simulink library "MPSV"  (R2025b)
settings: Solver=VariableStepAuto  StartTime=0.0  StopTime=10.0  RelTol=1e-3
undefined symbols (not defined in the file or in its folder): cost, errorCode, goalReached, isFeasible, numberOfPerformedIterations, numPoses, outOfNodes, path, timestampOfComputationUTC
libraries: simulink x31, $bdroot x11, etargetslib x5
(part 1 of 3)
settings Model: Creator=damerius  LastModifiedBy=damerius
settings SolverCC: AlgebraicLoopSolver=TrustRegion
settings OptimizationCC: ReuseModelBlockBuffer=off
settings DebuggingCC: UnconnectedInputMsg=warning  UnconnectedOutputMsg=warning  UnconnectedLineMsg=warning
settings ModelReferenceCC: EnableRefExpFcnMdlSchedulingChecks=on
settings RTWCC: GPUComputeCapability=3.5  DLArmComputeVersion=19.05

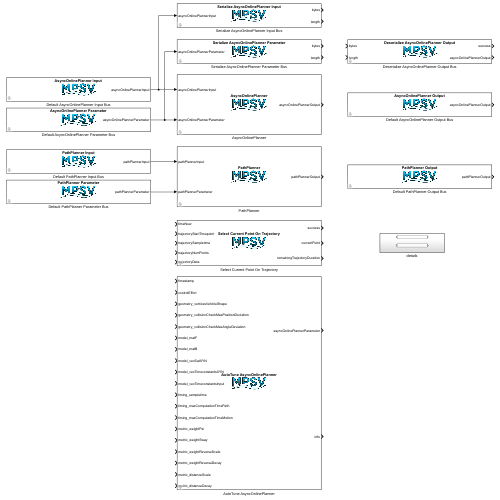
[thumbnail: Simulink's stored preview of the top-level diagram]
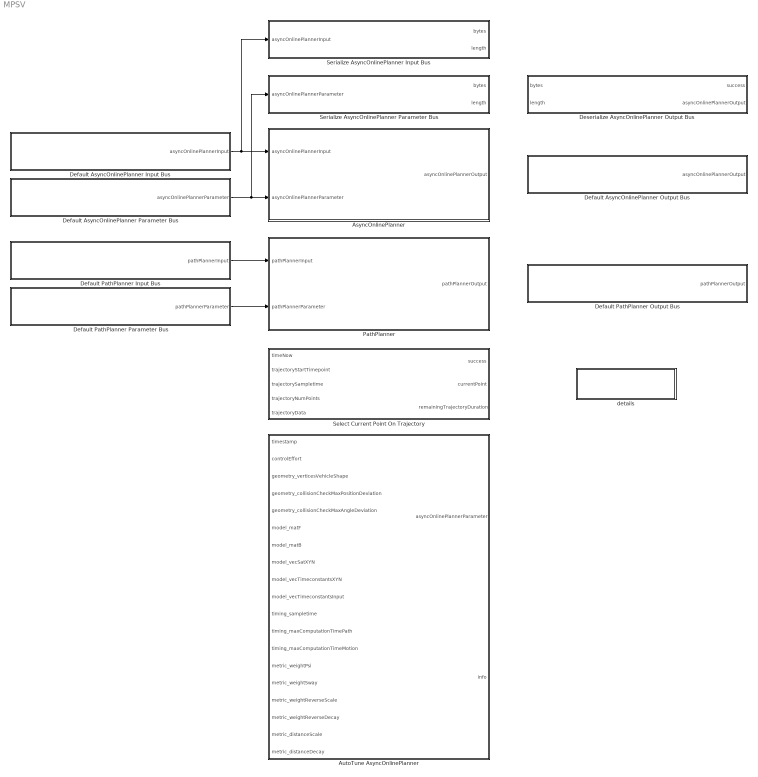
== system MPSV ==
  AsyncOnlinePlanner : Subsystem  mask{pathMaxNumNodes=200, pathMaxNumSamples=1000000, motionMaxNumNodes=200, motionMaxNumSamples=1000000, threadPriority=20, cpuCoreIDs=[], ompNumThreads=-1, ompDynamic=-1}
      mask prompts: pathMaxNumNodes "Maximum number of nodes for path planning (at least 2):"; pathMaxNumSamples "Maximum number of samples for path planning (at least 1):"; motionMaxNumNodes "Maximum number of nodes for motion planning (at least 2):"; motionMaxNumSamples "Maximum number of samples for path planning (at least 1):"; threadPriority "Thread priority (1: low, 99: high):"; cpuCoreIDs "CPU cores on which the thread is eligible to run, e.g. [0,1,2,3] ([] to ignore):"; ompNumThreads "OMP_NUM_THREADS (less than 1 to ignore):"; ompDynamic "OMP_DYNAMIC (-1 to ignore):"
      mask help:
      | Solve the online sequential motion planning problem in an asynchronous running parallel thread. For all kinds of timestamps, an arbitrary time source can be selected by the user. However, all times must be given in seconds and must be monotonically increasing.<br><br>
      |
      | <b>threadState</b><br>
      | The execution state of the asynchronous thread has the following enumeration:<br>
      | <table border="1" cellpadding="4" cellspacing="2">
      | <tr><th align="left">Value</th><th align="left">Name</th><th align="left">Description</th></tr>
      | <tr><td>0</td><td>offline</td><td>Thread has not been started.</td></tr>
      | <tr><td>1</td><td>standby</td><td>Thread is suspended and waits forever.</td></tr>
      | <tr><td>2</td><td>running</td><td>Thread solves motion planning problem.</td></tr>
      | </table>
      mask Help: eval('mpsv.OpenDocumentation(''library_asynconlineplanner.html'');');
      mask DialogControl DescGroupVar Prompt: MPSV - AsyncOnlinePlanner
      mask DialogControl Container4 Prompt: Memory Settings
      mask DialogControl Container2 Prompt: Path Planner
      mask DialogControl Container5 Prompt: Motion Planner
      mask DialogControl Container6 Prompt: Thread Settings
      mask DialogControl Container7 Prompt: Parallel Computing
      mask Display:
      | % Get dimension of block
      | pos = get_param(gcb, 'Position');
      | width = pos(3) - pos(1);
      | height = pos(4) - pos(2);
      | 
      | % Set image to center of block
      | imgWidth = 93;
      | imgHeight = 32;
      | image('MPSV_Icon.svg', [0.5*(width-imgWidth),0.5*(height-imgHeight),imgWidth,imgHeight]);
      | 
      | % Block title
      | text(0.5*width,0.5*(height+imgHeight)+2, '{\bfAsyncOnlinePlanner}','horizontalAlignment','center','verticalAlignment','bottom','texmode','on');
  AutoTune AsyncOnlinePlanner : Subsystem  mask{timeoutInput=1, periodGoalSampling=30}
      mask prompts: timeoutInput "Timeout for input data to the solver (default is 1):"; periodGoalSampling "Goal sampling period (default is 30):"
      mask help:
      | Calculate all tuning parameters for the MPSV AsyncOnlinePlanner based on given vehicle parameters and one intuitive tuning parameter. For more information take a look to the help page of mpsv.designer.AutoTune.<br><br>
      | <b>timestamp</b><br>
      | The timestamp to be set for the parameter data whenever at least one parameter changes.<br><br>
      | <b>controlEffort</b><br>
      | The amount of control effort in range (0,1] used to drive the vehicle in a steady-state in longitudinal direction.<br>
      mask DialogControl DescGroupVar Prompt: MPSV - AutoTune AsyncOnlinePlanner
      mask Display:
      | % Get dimension of block
      | pos = get_param(gcb, 'Position');
      | width = pos(3) - pos(1);
      | height = pos(4) - pos(2);
      | 
      | % Set image to center of block
      | imgWidth = 93;
      | imgHeight = 32;
      | image('MPSV_Icon.svg', [0.5*(width-imgWidth),0.5*(height-imgHeight),imgWidth,imgHeight]);
      | 
      | % Block title
      | text(0.5*width,0.5*(height+imgHeight)+2, '{\bfAutoTune AsyncOnlinePlanner}','horizontalAlignment','center','verticalAlignment','bottom','texmode','on');
  Default AsyncOnlinePlanner Input Bus : Subsystem
      mask help: Construct a default input bus for the AsyncOnlinePlanner. All values are set to zero.
      mask Help: eval('mpsv.OpenDocumentation(''library_asynconlineplannerinput.html'');');
      mask DialogControl DescGroupVar Prompt: MPSV - Default AsyncOnlinePlanner Input Bus
      mask Display:
      | % Get dimension of block
      | pos = get_param(gcb, 'Position');
      | width = pos(3) - pos(1);
      | height = pos(4) - pos(2);
      | 
      | % Set image to center of block
      | imgWidth = 93;
      | imgHeight = 32;
      | image('MPSV_Icon.svg', [0.5*(width-imgWidth),0.5*(height-imgHeight),imgWidth,imgHeight]);
      | 
      | % Block title
      | text(0.5*width,0.5*(height+imgHeight)+2, '{\bfAsyncOnlinePlanner Input}','horizontalAlignment','center','verticalAlignment','bottom','texmode','on');
  Default AsyncOnlinePlanner Output Bus : Subsystem
      mask help: Construct a default output bus for the AsyncOnlinePlanner. All values are set to zero.
      mask Help: eval('mpsv.OpenDocumentation(''library_asynconlineplanneroutput.html'');');
      mask DialogControl DescGroupVar Prompt: MPSV - Default AsyncOnlinePlanner Output Bus
      mask Display:
      | % Get dimension of block
      | pos = get_param(gcb, 'Position');
      | width = pos(3) - pos(1);
      | height = pos(4) - pos(2);
      | 
      | % Set image to center of block
      | imgWidth = 93;
      | imgHeight = 32;
      | image('MPSV_Icon.svg', [0.5*(width-imgWidth),0.5*(height-imgHeight),imgWidth,imgHeight]);
      | 
      | % Block title
      | text(0.5*width,0.5*(height+imgHeight)+2, '{\bfAsyncOnlinePlanner Output}','horizontalAlignment','center','verticalAlignment','bottom','texmode','on');
  Default AsyncOnlinePlanner Parameter Bus : Subsystem
      mask help: Construct a default parameter bus for the AsyncOnlinePlanner. All values are set to valid default values.
      mask Help: eval('mpsv.OpenDocumentation(''library_asynconlineplannerparameter.html'');');
      mask DialogControl DescGroupVar Prompt: MPSV - Default AsyncOnlinePlanner Parameter Bus
      mask Display:
      | % Get dimension of block
      | pos = get_param(gcb, 'Position');
      | width = pos(3) - pos(1);
      | height = pos(4) - pos(2);
      | 
      | % Set image to center of block
      | imgWidth = 93;
      | imgHeight = 32;
      | image('MPSV_Icon.svg', [0.5*(width-imgWidth),0.5*(height-imgHeight),imgWidth,imgHeight]);
      | 
      | % Block title
      | text(0.5*width,0.5*(height+imgHeight)+2, '{\bfAsyncOnlinePlanner Parameter}','horizontalAlignment','center','verticalAlignment','bottom','texmode','on');
  Default PathPlanner Input Bus : Subsystem
      mask help: Construct a default input bus for the PathPlanner. All values are set to zero.
      mask Help: eval('mpsv.OpenDocumentation(''library_pathplannerinput.html'');');
      mask DialogControl DescGroupVar Prompt: MPSV - Default PathPlanner Input Bus
      mask Display:
      | % Get dimension of block
      | pos = get_param(gcb, 'Position');
      | width = pos(3) - pos(1);
      | height = pos(4) - pos(2);
      | 
      | % Set image to center of block
      | imgWidth = 93;
      | imgHeight = 32;
      | image('MPSV_Icon.svg', [0.5*(width-imgWidth),0.5*(height-imgHeight),imgWidth,imgHeight]);
      | 
      | % Block title
      | text(0.5*width,0.5*(height+imgHeight)+2, '{\bfPathPlanner Input}','horizontalAlignment','center','verticalAlignment','bottom','texmode','on');
  Default PathPlanner Output Bus : Subsystem
      mask help: Construct a default output bus for the PathPlanner. All values are set to zero.
      mask Help: eval('mpsv.OpenDocumentation(''library_pathplanneroutput.html'');');
      mask DialogControl DescGroupVar Prompt: MPSV - Default PathPlanner Output Bus
      mask Display:
      | % Get dimension of block
      | pos = get_param(gcb, 'Position');
      | width = pos(3) - pos(1);
      | height = pos(4) - pos(2);
      | 
      | % Set image to center of block
      | imgWidth = 93;
      | imgHeight = 32;
      | image('MPSV_Icon.svg', [0.5*(width-imgWidth),0.5*(height-imgHeight),imgWidth,imgHeight]);
      | 
      | % Block title
      | text(0.5*width,0.5*(height+imgHeight)+2, '{\bfPathPlanner Output}','horizontalAlignment','center','verticalAlignment','bottom','texmode','on');
  Default PathPlanner Parameter Bus : Subsystem
      mask help: Construct a default parameter bus for the PathPlanner. All values are set to valid default values.
      mask Help: eval('mpsv.OpenDocumentation(''library_pathplannerparameter.html'');');
      mask DialogControl DescGroupVar Prompt: MPSV - Default PathPlanner Parameter Bus
      mask Display:
      | % Get dimension of block
      | pos = get_param(gcb, 'Position');
      | width = pos(3) - pos(1);
      | height = pos(4) - pos(2);
      | 
      | % Set image to center of block
      | imgWidth = 93;
      | imgHeight = 32;
      | image('MPSV_Icon.svg', [0.5*(width-imgWidth),0.5*(height-imgHeight),imgWidth,imgHeight]);
      | 
      | % Block title
      | text(0.5*width,0.5*(height+imgHeight)+2, '{\bfPathPlanner Parameter}','horizontalAlignment','center','verticalAlignment','bottom','texmode','on');
  Deserialize AsyncOnlinePlanner Output Bus : Subsystem
      mask help: Deserialize an AsyncOnlinePlanner output bus from a binary representation.
      mask Help: eval('mpsv.OpenDocumentation(''library_deserializeasynconlineplanneroutput.html'');');
      mask DialogControl DescGroupVar Prompt: MPSV - Deserialize AsyncOnlinePlanner Output Bus
      mask Display:
      | % Get dimension of block
      | pos = get_param(gcb, 'Position');
      | width = pos(3) - pos(1);
      | height = pos(4) - pos(2);
      | 
      | % Set image to center of block
      | imgWidth = 93;
      | imgHeight = 32;
      | image('MPSV_Icon.svg', [0.5*(width-imgWidth),0.5*(height-imgHeight),imgWidth,imgHeight]);
      | 
      | % Block title
      | text(0.5*width,0.5*(height+imgHeight)+2, '{\bfDeserialize AsyncOnlinePlanner Output}','horizontalAlignment','center','verticalAlignment','bottom','texmode','on');
  PathPlanner : Subsystem  mask{maxNumNodes=200, maxNumSamples=1000000}
      mask prompts: maxNumNodes "Maximum number of nodes (at least 2):"; maxNumSamples "Maximum number of samples (at least 1):"
      mask help: Solve the path planning problem. The computation time to be used by the planner is set via the parameter input. For all kinds of timestamps, an arbitrary time source can be selected by the user. However, all times must be given in seconds and must be monotonically increasing.
      mask Help: eval('mpsv.OpenDocumentation(''library_pathplanner.html'');');
      mask DialogControl DescGroupVar Prompt: Path Planner
      mask DialogControl ParameterGroupVar Prompt: Memory Settings
      mask Display:
      | % Get dimension of block
      | pos = get_param(gcb, 'Position');
      | width = pos(3) - pos(1);
      | height = pos(4) - pos(2);
      | 
      | % Set image to center of block
      | imgWidth = 93;
      | imgHeight = 32;
      | image('MPSV_Icon.svg', [0.5*(width-imgWidth),0.5*(height-imgHeight),imgWidth,imgHeight]);
      | 
      | % Block title
      | text(0.5*width,0.5*(height+imgHeight)+2, '{\bfPathPlanner}','horizontalAlignment','center','verticalAlignment','bottom','texmode','on');
  Select Current Point On Trajectory : Subsystem
      mask help:
      | Select the current point on a given trajectory for a given timepoint. An arbitrary time source can be selected by the user. However, all times must be given in seconds and must be monotonically increasing.<br><br>
      |
      | <b>timeNow</b><br>
      | The current timepoint to be used to query the point on the given trajectory.
      | <br><br>
      |
      | <b>trajectoryStartTimepoint</b><br>
      | The timepoint that indicates the first data point of the trajectory.
      | <br><br>
      |
      | <b>trajectorySampletime</b><br>
      | The temporal distance between two points of the trajectory.
      | <br><br>
      |
      | <b>trajectoryNumPoints</b><br>
      | The number of points to be considered from the trajectoryData matrix.
      | <br><br>
      |
      | <b>trajectoryData</b><br>
      | A 12-by-500 matrix containing 500 points of the trajectory, where each point represents the state-input-vector [x; y; psi; u; v; r; X; Y; N; Xc; Yc; Nc].
      | <br><br>
      |
      | <b>success</b><br>
      | True if timeNow lies within the temporal range of the trajectory and a point can be selected, false otherwise.
      | <br><br>
      |
      | <b>currentPoint</b><br>
      | A bus containing the linear interpolated state values and the zero-order hold input values.
      | <br><br>
      |
      | <b>remainingTrajectoryDuration</b><br>
      | Time from timeNow to the end of the trajectory.
      mask Help: eval('mpsv.OpenDocumentation(''library_selectcurrentpointontrajectory.html'');');
      mask DialogControl DescGroupVar Prompt: MPSV - Select Current Point On Trajectory
      mask Display:
      | % Get dimension of block
      | pos = get_param(gcb, 'Position');
      | width = pos(3) - pos(1);
      | height = pos(4) - pos(2);
      | 
      | % Set image to center of block
      | imgWidth = 93;
      | imgHeight = 32;
      | image('MPSV_Icon.svg', [0.5*(width-imgWidth),0.5*(height-imgHeight),imgWidth,imgHeight]);
      | 
      | % Block title
      | text(0.5*width,0.5*(height+imgHeight)+2, '{\bfSelect Current Point On Trajectory}','horizontalAlignment','center','verticalAlignment','bottom','texmode','on');
  Serialize AsyncOnlinePlanner Input Bus : Subsystem
      mask help: Serialize an AsyncOnlinePlanner input bus to a binary representation.
      mask Help: eval('mpsv.OpenDocumentation(''library_serializeasynconlineplannerinput.html'');');
      mask DialogControl DescGroupVar Prompt: MPSV - Serialize AsyncOnlinePlanner Input Bus
      mask Display:
      | % Get dimension of block
      | pos = get_param(gcb, 'Position');
      | width = pos(3) - pos(1);
      | height = pos(4) - pos(2);
      | 
      | % Set image to center of block
      | imgWidth = 93;
      | imgHeight = 32;
      | image('MPSV_Icon.svg', [0.5*(width-imgWidth),0.5*(height-imgHeight),imgWidth,imgHeight]);
      | 
      | % Block title
      | text(0.5*width,0.5*(height+imgHeight)+2, '{\bfSerialize AsyncOnlinePlanner Input}','horizontalAlignment','center','verticalAlignment','bottom','texmode','on');
  Serialize AsyncOnlinePlanner Parameter Bus : Subsystem
      mask help: Serialize an AsyncOnlinePlanner parameter bus to a binary representation.
      mask Help: eval('mpsv.OpenDocumentation(''library_serializeasynconlineplannerparameter.html'');');
      mask DialogControl DescGroupVar Prompt: MPSV - Serialize AsyncOnlinePlanner Parameter Bus
      mask Display:
      | % Get dimension of block
      | pos = get_param(gcb, 'Position');
      | width = pos(3) - pos(1);
      | height = pos(4) - pos(2);
      | 
      | % Set image to center of block
      | imgWidth = 93;
      | imgHeight = 32;
      | image('MPSV_Icon.svg', [0.5*(width-imgWidth),0.5*(height-imgHeight),imgWidth,imgHeight]);
      | 
      | % Block title
      | text(0.5*width,0.5*(height+imgHeight)+2, '{\bfSerialize AsyncOnlinePlanner Parameter}','horizontalAlignment','center','verticalAlignment','bottom','texmode','on');
  details : Subsystem
  wires:
  Default PathPlanner Input Bus/1(pathPlannerInput) -> PathPlanner/1(pathPlannerInput)
  Default AsyncOnlinePlanner Input Bus/1(asyncOnlinePlannerInput) -> Serialize AsyncOnlinePlanner Input Bus/1(asyncOnlinePlannerInput), AsyncOnlinePlanner/1(asyncOnlinePlannerInput)
  Default AsyncOnlinePlanner Parameter Bus/1(asyncOnlinePlannerParameter) -> Serialize AsyncOnlinePlanner Parameter Bus/1(asyncOnlinePlannerParameter), AsyncOnlinePlanner/2(asyncOnlinePlannerParameter)
  Default PathPlanner Parameter Bus/1(pathPlannerParameter) -> PathPlanner/2(pathPlannerParameter)

== system MPSV/AsyncOnlinePlanner ==
  asyncOnlinePlannerInput : Inport
  asyncOnlinePlannerParameter : Inport  Port=2
  Deserialize AsyncOnlinePlanner Output Bus : $bdroot/Deserialize AsyncOnlinePlanner Output Bus
  SFunctionMPSVAsynchronousOnlinePlanner : S-Function  FunctionName=SFunctionMPSVAsynchronousOnlinePlanner  Parameters=SParameter1, SParameter2, SParameter3, SParameter4, SParameter5, SParameter6, SParameter7, SParameter8, SParameter9  SFunctionDeploymentMode=off  EnableBusSupport=off  mask(Legacy Function){SFunctionSpec=void MPSV_AsynchronousOnlinePlannerStep(void* work1, uint8 y1[52907], uint8 u1[64193], uint8 u2[1917]), SParameter1=int16(pathMaxNumNodes), SParameter2=uint32(pathMaxNumSamples), SParameter3=int16(motionMaxNumNodes), SParameter4=uint32(motionMaxNumSamples), SParameter5=int32(threadPriority), SParameter6=int32(ompNumThreads), SParameter7=int32(ompDynamic), SParameter8=int32([reshape(cpuCoreIDs,[],1); -1]), SParameter9=uint32(numel(cpuCoreIDs)), ShowSpec=on}
      mask prompts: SParameter1 "P1:"; SParameter2 "P2:"; SParameter3 "P3:"; SParameter4 "P4:"; SParameter5 "P5:"; SParameter6 "P6:"; SParameter7 "P7:"; SParameter8 "P8:"; SParameter9 "P9:"; ShowSpec "Display function specification"
      mask help:
      | This block allows you to call the legacy functions specified by the following Legacy Code Tool definition:
      | def.SFunctionName = 'SFunctionMPSVAsynchronousOnlinePlanner';
      | def.OutputFcnSpec = 'void MPSV_AsynchronousOnlinePlannerStep(void* work1, uint8 y1[52907], uint8 u1[64193], uint8 u2[1917])';
      | def.StartFcnSpec = 'void MPSV_AsynchronousOnlinePlannerInitialize(void** work1, int16 p1, uint32 p2, int16 p3, uint32 p4, int32 p5, int32 p6, int32 p7, int32 p8[], uint32 p9)';
      | def.TerminateFcnSpec = 'void MPSV_AsynchronousOnlinePlannerTerminate(void* work1)';
      | def.HeaderFiles = {'MPSV_DriverAsynchronousOnlinePlanner.hpp'};
      | def.SourceFiles = {'MPSV_DriverAsynchronousOnlinePlanner.cpp', 'MPSV_WrapperAsynchronousOnlinePlanner.cpp'};
      | def.IncPaths = {'code'};
      | def.SrcPaths = {'code'};
      | def.Options.useTlcWithAccel = false;
      mask Help: <p>This block was generated automatically by the Legacy Code Tool. For detailed help on this tool, call<a href="matlab:legacy_code('help')"> legacy_code('help')</a>.</p>
      mask Callback ShowSpec:
      | if strcmp(get_param(gcbh, 'ShowSpec'), 'on')
      |   set_param(gcbh, 'MaskDisplay', sprintf('fprintf(''%s'');', get_param(gcbh, 'SFunctionSpec')));
      | else
      |   set_param(gcbh, 'MaskDisplay', sprintf('fprintf(''%s'');', get_param(gcbh, 'FunctionName')));
      | end
      mask Display: fprintf('void MPSV_AsynchronousOnlinePlannerStep(void* work1, uint8 y1[52907], uint8 u1[64193], uint8 u2[1917])');
  Serialize AsyncOnlinePlanner Input Bus : $bdroot/Serialize AsyncOnlinePlanner Input Bus
  Serialize AsyncOnlinePlanner Parameter Bus : $bdroot/Serialize AsyncOnlinePlanner Parameter Bus
  Terminator : Terminator
  Terminator1 : Terminator
  Terminator2 : Terminator
  Width : Width  DataType=uint32
  asyncOnlinePlannerOutput : Outport
  wires:
  asyncOnlinePlannerInput/1 -> Serialize AsyncOnlinePlanner Input Bus/1
  Deserialize AsyncOnlinePlanner Output Bus/2 -> asyncOnlinePlannerOutput/1
  asyncOnlinePlannerParameter/1 -> Serialize AsyncOnlinePlanner Parameter Bus/1
  SFunctionMPSVAsynchronousOnlinePlanner/1 -> Width/1, Deserialize AsyncOnlinePlanner Output Bus/1
  Serialize AsyncOnlinePlanner Input Bus/1 -> SFunctionMPSVAsynchronousOnlinePlanner/1
  Serialize AsyncOnlinePlanner Parameter Bus/1 -> SFunctionMPSVAsynchronousOnlinePlanner/2
  Serialize AsyncOnlinePlanner Input Bus/2 -> Terminator/1
  Serialize AsyncOnlinePlanner Parameter Bus/2 -> Terminator1/1
  Width/1 -> Deserialize AsyncOnlinePlanner Output Bus/2
  Deserialize AsyncOnlinePlanner Output Bus/1 -> Terminator2/1

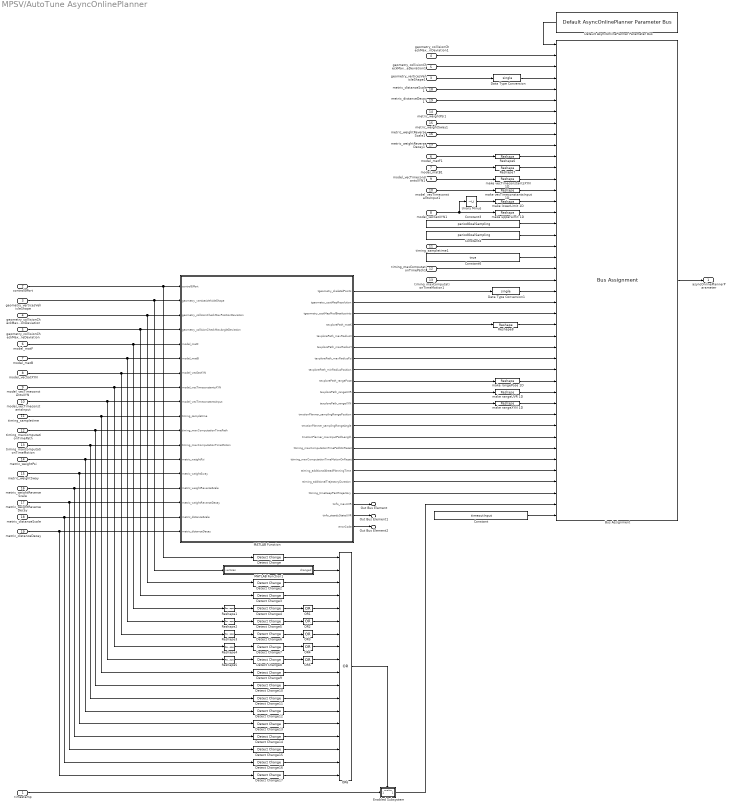
== system MPSV/AutoTune AsyncOnlinePlanner ==
  timestamp : Inport
  controlEffort : Inport  Port=2
  geometry_verticesVehicleShape : Inport  Port=3
  geometry_collisionCheckMaxPositionDeviation : Inport  Port=4
  geometry_collisionCheckMaxAngleDeviation : Inport  Port=5
  model_matF : Inport  Port=6
  model_matB : Inport  Port=7
  model_vecSatXYN : Inport  Port=8
  model_vecTimeconstantsXYN : Inport  Port=9
  model_vecTimeconstantsInput : Inport  Port=10
  timing_sampletime : Inport  Port=11
  timing_maxComputationTimePath : Inport  Port=12
  timing_maxComputationTimeMotion : Inport  Port=13
  metric_weightPsi : Inport  Port=14
  metric_weightSway : Inport  Port=15
  metric_weightReverseScale : Inport  Port=16
  metric_weightReverseDecay : Inport  Port=17
  metric_distanceScale : Inport  Port=18
  metric_distanceDecay : Inport  Port=19
  Bus Assignment : BusAssignment  AssignedSignals=sequentialPlanner.geometry.collisionCheckMaxPositionDeviation,sequentialPlanner.geometry.collisionCheckMaxAngleDeviation,sequentialPlanner.geometry.verticesVehicleShape,sequentialPlanner.costMap.distanceScale,sequentialPlanner.costMap.distanceDecay,sequentialPlanner.metric.weightPsi,sequentialPlanner.metric.weightSway,sequentialPlanner.metric.weightReverseScale,sequentialPlanner.metric.weightReverseDecay,sequentialPlanner.model.matF,sequentialPlanner.model.matB,sequentialPlanner.model.vecTimeconstantsXYN,sequentialPlanner.model.vecTimeconstantsInput,sequentialPlanner.model.lowerLimitXYN,sequentialPlanner.model.upperLimitXYN,sequentialPlanner.pathPlanner.periodGoalSampling,sequentialPlanner.motionPlanner.periodGoalSampling,sequentialPlanner.motionPlanner.sampletime,onlinePlanner.predictInitialStateOnReset,onlinePlanner.maxComputationTimePath,onlinePlanner.maxComputationTimeMotion,sequentialPlanner.geometry.skeletalPoints,sequentialPlanner.costMap.resolution,sequentialPlanner.costMap.modBreakpoints,sequentialPlanner.motionPlanner.controller.matK,sequentialPlanner.motionPlanner.controller.maxRadiusX,sequentialPlanner.motionPlanner.controller.maxRadiusY,sequentialPlanner.motionPlanner.controller.maxRadiusPsi,sequentialPlanner.motionPlanner.controller.minRadiusPosition,sequentialPlanner.motionPlanner.regionOfAttraction.rangePose,sequentialPlanner.motionPlanner.regionOfAttraction.rangeUVR,sequentialPlanner.motionPlanner.regionOfAttraction.rangeXYN,sequentialPlanner.motionPlanner.samplingRangePosition,sequentialPlanner.motionPlanner.samplingRangeAngle,sequentialPlanner.motionPlanner.maxInputPathLength,onlinePlanner.maxComputationTimePathOnReset,onlinePlanner.maxComputationTimeMotionOnReset,onlinePlanner.additionalAheadPlanningTime,onlinePlanner.additionalTrajectoryDuration,onlinePlanner.timeKeepPastTrajectory,timestamp,timeoutInput
  Constant : Constant  Value=timeoutInput  OutDataTypeStr=double
  Constant3 : Constant  Value=periodGoalSampling  OutDataTypeStr=uint32
  Constant4 : Constant  Value=periodGoalSampling  OutDataTypeStr=uint32
  Constant6 : Constant  Value=true  OutDataTypeStr=boolean
  Data Type Conversion : DataTypeConversion  OutDataTypeStr=single  SaturateOnIntegerOverflow=off  RndMeth=Floor
  Data Type Conversion1 : DataTypeConversion  OutDataTypeStr=single  SaturateOnIntegerOverflow=off  RndMeth=Floor
  Default AsyncOnlinePlanner Parameter Bus : $bdroot/Default AsyncOnlinePlanner Parameter Bus
  Detect Change{,2..17} (17 alike) : simulink/Logic and Bit Operations/Detect Change  vinit=0  OutDataTypeStr=boolean
  Enabled Subsystem : Subsystem  TreatAsAtomicUnit=on
  MATLAB Function : MATLAB Function  TreatAsAtomicUnit=on
  MATLAB Function1 : MATLAB Function  TreatAsAtomicUnit=on
  OR{1..5} (5 alike) : Logic  Operator=OR  Inputs=1  AllPortsSameDT=off  OutDataTypeStr=boolean
  OR6 : Logic  Operator=OR  Inputs=18  AllPortsSameDT=off  OutDataTypeStr=boolean
  Reshape{1..5} (5 alike) : Reshape  OutputDimensionality=Column vector (2-D)
  Reshape6 : Reshape  OutputDimensionality=Customize  OutputDimensions=[3,12]
  Reshape7 : Reshape  OutputDimensionality=Customize  OutputDimensions=[3,3]
  Reshape8 : Reshape  OutputDimensionality=Customize  OutputDimensions=[3,12]
  Unary Minus : UnaryMinus
  geometry_collisionCheckMaxAngleDeviation1 : InportShadow  Port=5
  geometry_collisionCheckMaxPositionDeviation1 : InportShadow  Port=4
  geometry_verticesVehicleShape1 : InportShadow  Port=3
  make lowerLimit 1D : Reshape
  make rangePose 1D : Reshape
  make rangeUVR 1D : Reshape
  make rangeXYN 1D : Reshape
  make upperLimit 1D : Reshape
  make vecTimeconstantsInput 1D : Reshape
  make vecTimeconstantsXYN 1D : Reshape
  metric_distanceDecay1 : InportShadow  Port=19
  metric_distanceScale1 : InportShadow  Port=18
  metric_weightPsi1 : InportShadow  Port=14
  metric_weightReverseDecay1 : InportShadow  Port=17
  metric_weightReverseScale1 : InportShadow  Port=16
  metric_weightSway1 : InportShadow  Port=15
  model_matB1 : InportShadow  Port=7
  model_matF1 : InportShadow  Port=6
  model_vecSatXYN1 : InportShadow  Port=8
  model_vecTimeconstantsInput1 : InportShadow  Port=10
  model_vecTimeconstantsXYN1 : InportShadow  Port=9
  timing_maxComputationTimeMotion1 : InportShadow  Port=13
  timing_maxComputationTimePath1 : InportShadow  Port=12
  timing_sampletime1 : InportShadow  Port=11
  asyncOnlinePlannerParameter : Outport
  Out Bus Element : Outport  Port=2  PortName=info  Element=modelMaxUVR
  Out Bus Element1 : Outport  Port=2  PortName=info  Element=modelSteadyStateUVR
  Out Bus Element2 : Outport  Port=2  PortName=info  Element=errorCode
  wires:
  MATLAB Function1/1(changed) -> OR6/2
  Reshape5/1 -> Detect Change8/1
  Reshape4/1 -> Detect Change7/1
  Reshape3/1 -> Detect Change6/1
  Reshape2/1 -> Detect Change5/1
  Reshape1/1 -> Detect Change4/1
  Detect Change17/1 -> OR6/18
  Detect Change16/1 -> OR6/17
  Detect Change15/1 -> OR6/16
  Detect Change14/1 -> OR6/15
  Detect Change13/1 -> OR6/14
  Detect Change12/1 -> OR6/13
  Detect Change11/1 -> OR6/12
  Detect Change10/1 -> OR6/11
  Detect Change9/1 -> OR6/10
  OR5/1 -> OR6/9
  OR4/1 -> OR6/8
  OR3/1 -> OR6/7
  OR2/1 -> OR6/6
  OR1/1 -> OR6/5
  Detect Change3/1 -> OR6/4
  Detect Change2/1 -> OR6/3
  Detect Change/1 -> OR6/1
  Detect Change8/1 -> OR5/1
  Detect Change6/1 -> OR3/1
  Detect Change7/1 -> OR4/1
  Detect Change5/1 -> OR2/1
  Detect Change4/1 -> OR1/1
  metric_distanceDecay/1 -> Detect Change17/1, MATLAB Function/18(metric_distanceDecay)
  metric_distanceScale/1 -> Detect Change16/1, MATLAB Function/17(metric_distanceScale)
  model_vecTimeconstantsInput/1 -> Reshape5/1, MATLAB Function/9(model_vecTimeconstantsInput)
  timing_sampletime/1 -> Detect Change9/1, MATLAB Function/10(timing_sampletime)
  timing_maxComputationTimeMotion/1 -> Detect Change11/1, MATLAB Function/12(timing_maxComputationTimeMotion)
  timing_maxComputationTimePath/1 -> Detect Change10/1, MATLAB Function/11(timing_maxComputationTimePath)
  metric_weightReverseScale/1 -> Detect Change14/1, MATLAB Function/15(metric_weightReverseScale)
  metric_weightReverseDecay/1 -> Detect Change15/1, MATLAB Function/16(metric_weightReverseDecay)
  metric_weightSway/1 -> Detect Change13/1, MATLAB Function/14(metric_weightSway)
  metric_weightPsi/1 -> Detect Change12/1, MATLAB Function/13(metric_weightPsi)
  model_matF/1 -> Reshape1/1, MATLAB Function/5(model_matF)
  model_matB/1 -> Reshape2/1, MATLAB Function/6(model_matB)
  model_vecTimeconstantsXYN/1 -> Reshape4/1, MATLAB Function/8(model_vecTimeconstantsXYN)
  model_vecSatXYN/1 -> Reshape3/1, MATLAB Function/7(model_vecSatXYN)
  geometry_collisionCheckMaxPositionDeviation/1 -> Detect Change2/1, MATLAB Function/3(geometry_collisionCheckMaxPositionDeviation)
  geometry_collisionCheckMaxAngleDeviation/1 -> Detect Change3/1, MATLAB Function/4(geometry_collisionCheckMaxAngleDeviation)
  geometry_verticesVehicleShape/1 -> MATLAB Function1/1(vertices), MATLAB Function/2(geometry_verticesVehicleShape)
  controlEffort/1 -> Detect Change/1, MATLAB Function/1(controlEffort)
  geometry_verticesVehicleShape1/1 -> Data Type Conversion/1
  Constant6/1 -> Bus Assignment/20
  model_vecTimeconstantsXYN1/1 -> make vecTimeconstantsXYN 1D/1
  model_matB1/1 -> Reshape7/1
  make rangeXYN 1D/1 -> Bus Assignment/33
  MATLAB Function/15(ttiming_maxComputationTimePathOnReset) -> Bus Assignment/37
  MATLAB Function/5(texplorePath_maxRadiusX) -> Bus Assignment/27
  OR6/1 -> Enabled Subsystem/Enable
  timing_sampletime1/1 -> Bus Assignment/19
  MATLAB Function/4(texplorePath_matK) -> Reshape8/1
  MATLAB Function/18(ttiming_additionalTrajectoryDuration) -> Bus Assignment/40
  model_vecSatXYN1/1 -> Unary Minus/1, make upperLimit 1D/1
  make rangePose 1D/1 -> Bus Assignment/31
  Data Type Conversion1/1 -> Bus Assignment/23
  MATLAB Function/19(ttiming_timeKeepPastTrajectory) -> Bus Assignment/41
  MATLAB Function/9(texplorePath_rangePose) -> make rangePose 1D/1
  MATLAB Function/17(ttiming_additionalAheadPlanningTime) -> Bus Assignment/39
  Reshape6/1 -> Bus Assignment/11
  Reshape7/1 -> Bus Assignment/12
  make rangeUVR 1D/1 -> Bus Assignment/32
  model_vecTimeconstantsInput1/1 -> make vecTimeconstantsInput 1D/1
  Unary Minus/1 -> make lowerLimit 1D/1
  timestamp/1 -> Enabled Subsystem/1(In1)
  make vecTimeconstantsInput 1D/1 -> Bus Assignment/14
  metric_distanceDecay1/1 -> Bus Assignment/6
  make upperLimit 1D/1 -> Bus Assignment/16
  MATLAB Function/1(tgeometry_skeletalPoints) -> Data Type Conversion1/1
  make lowerLimit 1D/1 -> Bus Assignment/15
  timing_maxComputationTimeMotion1/1 -> Bus Assignment/22
  Constant4/1 -> Bus Assignment/18
  model_matF1/1 -> Reshape6/1
  metric_weightSway1/1 -> Bus Assignment/8
  make vecTimeconstantsXYN 1D/1 -> Bus Assignment/13
  timing_maxComputationTimePath1/1 -> Bus Assignment/21
  Reshape8/1 -> Bus Assignment/26
  MATLAB Function/14(tmotionPlanner_maxInputPathLength) -> Bus Assignment/36
  MATLAB Function/10(texplorePath_rangeUVR) -> make rangeUVR 1D/1
  Constant3/1 -> Bus Assignment/17
  MATLAB Function/16(ttiming_maxComputationTimeMotionOnReset) -> Bus Assignment/38
  Enabled Subsystem/1(Out1) -> Bus Assignment/42
  MATLAB Function/11(texplorePath_rangeXYN) -> make rangeXYN 1D/1
  metric_weightPsi1/1 -> Bus Assignment/7
  Data Type Conversion/1 -> Bus Assignment/4
  metric_distanceScale1/1 -> Bus Assignment/5
  Default AsyncOnlinePlanner Parameter Bus/1 -> Bus Assignment/1
  geometry_collisionCheckMaxPositionDeviation1/1 -> Bus Assignment/2
  geometry_collisionCheckMaxAngleDeviation1/1 -> Bus Assignment/3
  MATLAB Function/3(tgeometry_costMapModBreakpoints) -> Bus Assignment/25
  MATLAB Function/2(tgeometry_costMapResolution) -> Bus Assignment/24
  metric_weightReverseScale1/1 -> Bus Assignment/9
  metric_weightReverseDecay1/1 -> Bus Assignment/10
  MATLAB Function/12(tmotionPlanner_samplingRangePosition) -> Bus Assignment/34
  MATLAB Function/13(tmotionPlanner_samplingRangeAngle) -> Bus Assignment/35
  MATLAB Function/6(texplorePath_maxRadiusY) -> Bus Assignment/28
  MATLAB Function/7(texplorePath_maxRadiusPsi) -> Bus Assignment/29
  MATLAB Function/8(texplorePath_minRadiusPosition) -> Bus Assignment/30
  Bus Assignment/1 -> asyncOnlinePlannerParameter/1
  Constant/1 -> Bus Assignment/43
  MATLAB Function/20(tinfo_maxUVR) -> Out Bus Element/1
  MATLAB Function/21(tinfo_steadyStateUVR) -> Out Bus Element1/1
  MATLAB Function/22(errorCode) -> Out Bus Element2/1

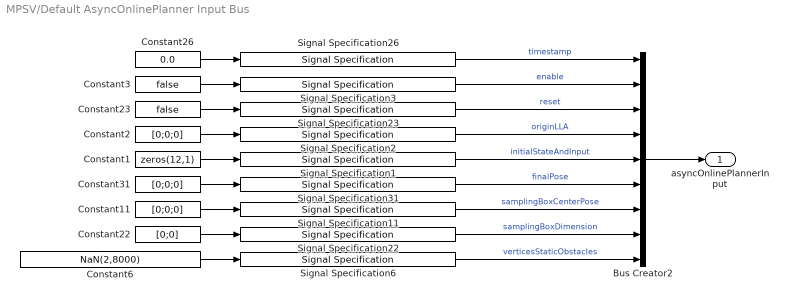
== system MPSV/Default AsyncOnlinePlanner Input Bus ==
  Bus Creator2 : BusCreator  Inputs=9
  Constant1 : Constant  Value=zeros(12,1)  OutDataTypeStr=double
  Constant11 : Constant  Value=[0;0;0]  OutDataTypeStr=double
  Constant2 : Constant  Value=[0;0;0]  OutDataTypeStr=double
  Constant22 : Constant  Value=[0;0]  OutDataTypeStr=double
  Constant23 : Constant  Value=false  OutDataTypeStr=boolean
  Constant26 : Constant  Value=0.0  OutDataTypeStr=double
  Constant3 : Constant  Value=false  OutDataTypeStr=boolean
  Constant31 : Constant  Value=[0;0;0]  OutDataTypeStr=double
  Constant6 : Constant  Value=NaN(2,8000)  OutDataTypeStr=single
  Signal Specification1 : SignalSpecification  OutDataTypeStr=double  Dimensions=12
  Signal Specification11 : SignalSpecification  OutDataTypeStr=double  Dimensions=3
  Signal Specification2 : SignalSpecification  OutDataTypeStr=double  Dimensions=3
  Signal Specification22 : SignalSpecification  OutDataTypeStr=double  Unit=m  Dimensions=2
  Signal Specification23 : SignalSpecification  OutDataTypeStr=boolean  Dimensions=1
  Signal Specification26 : SignalSpecification  OutDataTypeStr=double  Unit=s  Dimensions=1
  Signal Specification3 : SignalSpecification  OutDataTypeStr=boolean  Dimensions=1
  Signal Specification31 : SignalSpecification  OutDataTypeStr=double  Dimensions=3
  Signal Specification6 : SignalSpecification  OutDataTypeStr=single  Unit=m  Dimensions=[2,8000]
  asyncOnlinePlannerInput : Outport
  wires:
  Constant22/1 -> Signal Specification22/1
  Constant11/1 -> Signal Specification11/1
  Constant6/1 -> Signal Specification6/1
  Constant2/1 -> Signal Specification2/1
  Constant23/1 -> Signal Specification23/1
  Signal Specification23/1 -> Bus Creator2/3  "reset"
  Constant26/1 -> Signal Specification26/1
  Signal Specification26/1 -> Bus Creator2/1  "timestamp"
  Constant1/1 -> Signal Specification1/1
  Signal Specification1/1 -> Bus Creator2/5  "initialStateAndInput"
  Constant31/1 -> Signal Specification31/1
  Signal Specification31/1 -> Bus Creator2/6  "finalPose"
  Signal Specification2/1 -> Bus Creator2/4  "originLLA"
  Signal Specification11/1 -> Bus Creator2/7  "samplingBoxCenterPose"
  Signal Specification22/1 -> Bus Creator2/8  "samplingBoxDimension"
  Signal Specification6/1 -> Bus Creator2/9  "verticesStaticObstacles"
  Bus Creator2/1 -> asyncOnlinePlannerInput/1
  Constant3/1 -> Signal Specification3/1
  Signal Specification3/1 -> Bus Creator2/2  "enable"

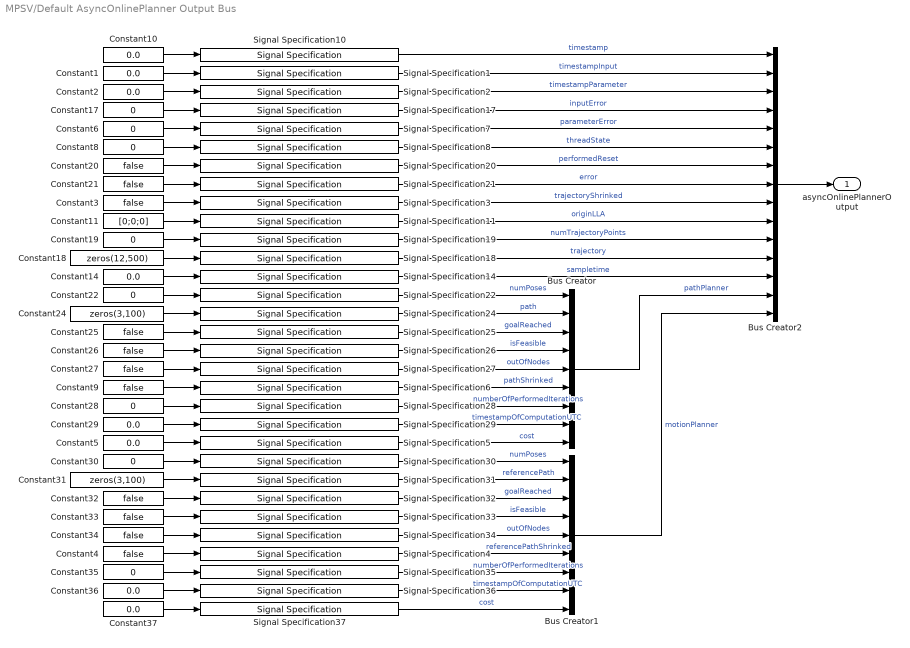
== system MPSV/Default AsyncOnlinePlanner Output Bus ==
  Bus Creator : BusCreator  Inputs=9
  Bus Creator1 : BusCreator  Inputs=9
  Bus Creator2 : BusCreator  Inputs=15
  Constant{1..2,5,10,14,29,36..37} (8 alike) : Constant  Value=0.0  OutDataTypeStr=double
  Constant11 : Constant  Value=[0;0;0]  OutDataTypeStr=double
  Constant17 : Constant  Value=0  OutDataTypeStr=uint8
  Constant18 : Constant  Value=zeros(12,500)  OutDataTypeStr=double
  Constant19 : Constant  Value=0  OutDataTypeStr=uint16
  Constant{3..4,9,20..21,25..27,32..34} (11 alike) : Constant  Value=false  OutDataTypeStr=boolean
  Constant22 : Constant  Value=0  OutDataTypeStr=uint16
  Constant24 : Constant  Value=zeros(3,100)  OutDataTypeStr=double
  Constant28 : Constant  Value=0  OutDataTypeStr=uint32
  Constant30 : Constant  Value=0  OutDataTypeStr=uint16
  Constant31 : Constant  Value=zeros(3,100)  OutDataTypeStr=double
  Constant35 : Constant  Value=0  OutDataTypeStr=uint32
  Constant6 : Constant  Value=0  OutDataTypeStr=uint8
  Constant8 : Constant  Value=0  OutDataTypeStr=uint8
  Signal Specification{1..2,10,14,29,36} (6 alike) : SignalSpecification  OutDataTypeStr=double  Unit=s  Dimensions=1
  Signal Specification11 : SignalSpecification  OutDataTypeStr=double  Dimensions=3
  Signal Specification17 : SignalSpecification  OutDataTypeStr=uint8  Dimensions=1
  Signal Specification18 : SignalSpecification  OutDataTypeStr=double  Dimensions=[12,500]
  Signal Specification19 : SignalSpecification  OutDataTypeStr=uint16  Dimensions=1
  Signal Specification{3..4,6,20..21,25..27,32..34} (11 alike) : SignalSpecification  OutDataTypeStr=boolean  Dimensions=1
  Signal Specification22 : SignalSpecification  OutDataTypeStr=uint16  Dimensions=1
  Signal Specification24 : SignalSpecification  OutDataTypeStr=double  Dimensions=[3,100]
  Signal Specification28 : SignalSpecification  OutDataTypeStr=uint32  Dimensions=1
  Signal Specification30 : SignalSpecification  OutDataTypeStr=uint16  Dimensions=1
  Signal Specification31 : SignalSpecification  OutDataTypeStr=double  Dimensions=[3,100]
  Signal Specification35 : SignalSpecification  OutDataTypeStr=uint32  Dimensions=1
  Signal Specification37 : SignalSpecification  OutDataTypeStr=double  Dimensions=1
  Signal Specification5 : SignalSpecification  OutDataTypeStr=double  Dimensions=1
  Signal Specification7 : SignalSpecification  OutDataTypeStr=uint8  Dimensions=1
  Signal Specification8 : SignalSpecification  OutDataTypeStr=uint8  Dimensions=1
  asyncOnlinePlannerOutput : Outport
  wires:
  Constant17/1 -> Signal Specification17/1
  Signal Specification1/1 -> Bus Creator2/2  "timestampInput"
  Bus Creator2/1 -> asyncOnlinePlannerOutput/1
  Signal Specification2/1 -> Bus Creator2/3  "timestampParameter"
  Constant8/1 -> Signal Specification8/1
  Signal Specification8/1 -> Bus Creator2/6  "threadState"
  Constant5/1 -> Signal Specification5/1
  Signal Specification5/1 -> Bus Creator/9  "cost"
  Constant10/1 -> Signal Specification10/1
  Signal Specification10/1 -> Bus Creator2/1  "timestamp"
  Constant11/1 -> Signal Specification11/1
  Signal Specification11/1 -> Bus Creator2/10  "originLLA"
  Constant14/1 -> Signal Specification14/1
  Constant18/1 -> Signal Specification18/1
  Constant19/1 -> Signal Specification19/1
  Signal Specification19/1 -> Bus Creator2/11  "numTrajectoryPoints"
  Signal Specification18/1 -> Bus Creator2/12  "trajectory"
  Signal Specification14/1 -> Bus Creator2/13  "sampletime"
  Constant20/1 -> Signal Specification20/1
  Signal Specification20/1 -> Bus Creator2/7  "performedReset"
  Constant21/1 -> Signal Specification21/1
  Signal Specification21/1 -> Bus Creator2/8  "error"
  Bus Creator/1 -> Bus Creator2/14  "pathPlanner"
  Constant22/1 -> Signal Specification22/1
  Signal Specification22/1 -> Bus Creator/1  "numPoses"
  Constant24/1 -> Signal Specification24/1
  Signal Specification24/1 -> Bus Creator/2  "path"
  Constant25/1 -> Signal Specification25/1
  Signal Specification25/1 -> Bus Creator/3  "goalReached"
  Constant26/1 -> Signal Specification26/1
  Signal Specification26/1 -> Bus Creator/4  "isFeasible"
  Constant27/1 -> Signal Specification27/1
  Signal Specification27/1 -> Bus Creator/5  "outOfNodes"
  Constant28/1 -> Signal Specification28/1
  Signal Specification28/1 -> Bus Creator/7  "numberOfPerformedIterations"
  Constant29/1 -> Signal Specification29/1
  Signal Specification29/1 -> Bus Creator/8  "timestampOfComputationUTC"
  Signal Specification36/1 -> Bus Creator1/8  "timestampOfComputationUTC"
  Constant36/1 -> Signal Specification36/1
  Signal Specification35/1 -> Bus Creator1/7  "numberOfPerformedIterations"
  Constant35/1 -> Signal Specification35/1
  Signal Specification34/1 -> Bus Creator1/5  "outOfNodes"
  Constant34/1 -> Signal Specification34/1
  Signal Specification33/1 -> Bus Creator1/4  "isFeasible"
  Constant33/1 -> Signal Specification33/1
  Signal Specification32/1 -> Bus Creator1/3  "goalReached"
  Constant32/1 -> Signal Specification32/1
  Signal Specification31/1 -> Bus Creator1/2  "referencePath"
  Constant31/1 -> Signal Specification31/1
  Signal Specification30/1 -> Bus Creator1/1  "numPoses"
  Constant30/1 -> Signal Specification30/1
  Signal Specification37/1 -> Bus Creator1/9  "cost"
  Constant37/1 -> Signal Specification37/1
  Bus Creator1/1 -> Bus Creator2/15  "motionPlanner"
  Constant1/1 -> Signal Specification1/1
  Constant2/1 -> Signal Specification2/1
  Signal Specification3/1 -> Bus Creator2/9  "trajectoryShrinked"
  Constant3/1 -> Signal Specification3/1
  Constant4/1 -> Signal Specification4/1
  Signal Specification4/1 -> Bus Creator1/6  "referencePathShrinked"
  Constant9/1 -> Signal Specification6/1
  Signal Specification6/1 -> Bus Creator/6  "pathShrinked"
  Constant6/1 -> Signal Specification7/1
  Signal Specification7/1 -> Bus Creator2/5  "parameterError"
  Signal Specification17/1 -> Bus Creator2/4  "inputError"
